simulink subsystem "Pharmacokinetic_Model"  (R2023b)
settings: Solver=VariableStepAuto  StartTime=0.0  StopTime=10.0  RelTol=1e-3
values from neighbouring files (symbols this model uses):
  V_c = 10    [Project2024_params_Group3.m]
undefined symbols (not defined in the file or in its folder): gamma
settings Model: Creator=jamesyeh  LastModifiedBy=jamesyeh

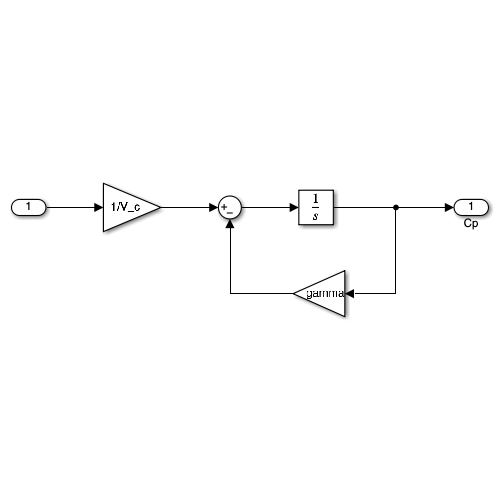
[thumbnail: Simulink's stored preview of the top-level diagram]
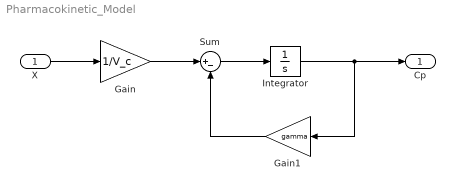
== system Pharmacokinetic_Model ==
  X : Inport
  Gain : Gain  Gain=1/V_c
  Gain1 : Gain  Gain=gamma
  Integrator : Integrator
  Sum : Sum  Inputs=|+-
  Cp : Outport
  wires:
  X/1 -> Gain/1
  Gain/1 -> Sum/1
  Sum/1 -> Integrator/1
  Integrator/1 -> Gain1/1, Cp/1
  Gain1/1 -> Sum/2
